simulink model "sim1"  (R2023a)
settings: Solver=VariableStepAuto  StartTime=0.0  StopTime=10.0  RelTol=1e-3
settings Model: Creator=hwayoungkim  LastModifiedBy=hwayoungkim

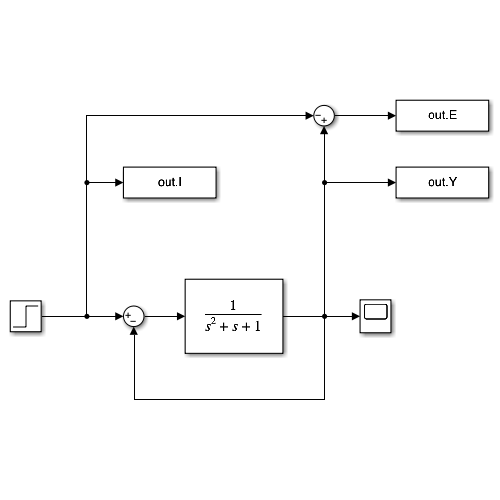
[thumbnail: Simulink's stored preview of the top-level diagram]
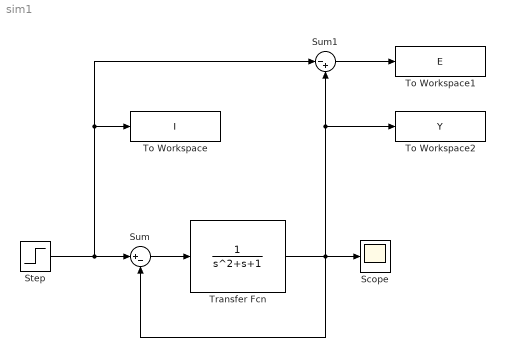
== system sim1 ==
  Scope : Scope
  Step : Step  Time=0  SampleTime=0
  Sum : Sum  Inputs=|+-
  Sum1 : Sum  Inputs=|-+
  To Workspace : ToWorkspace  VariableName=I  SaveFormat=Timeseries  SampleTime=-1
  To Workspace1 : ToWorkspace  VariableName=E  SaveFormat=Timeseries  SampleTime=-1
  To Workspace2 : ToWorkspace  VariableName=Y  SaveFormat=Timeseries  SampleTime=-1
  Transfer Fcn : TransferFcn  Denominator=[1 1 1]
  wires:
  Step/1 -> Sum/1, Sum1/1, To Workspace/1
  Transfer Fcn/1 -> Sum1/2, To Workspace2/1, Sum/2, Scope/1
  Sum1/1 -> To Workspace1/1
  Sum/1 -> Transfer Fcn/1
